simulink model "Aero_UltraStick25e"  (R2016b)
settings: Solver=VariableStepAuto  StartTime=0.0  StopTime=10.0  RelTol=1e-3
undefined symbols (not defined in the file or in its folder): AC
libraries: simulink x1
(part 2 of 2)

== system Aero_UltraStick25e/Yaw Moment Coefficient/Cnr*b//(2V) ==
  In : Inport
  2V : Gain  Gain=2  SaturateOnIntegerOverflow=on  OutDataTypeStr=Inherit: Same as input  ParamDataTypeStr=Inherit: Same as input
  Bus Selector4 : BusSelector  OutputSignals=AngVel.r_rps,WindAxesParams.alpha_rad,WindAxesParams.beta_rad,WindAxesParams.Vs_mps
  Cnr : Product
  Cnr Lookup : Interpolation_n-D  Table=AC.Aero.Cn.r_dat.data  InternalRulePriority=Speed
  Cnr*b/(2V) : Product  Inputs=**/  SaturateOnIntegerOverflow=on  RndMeth=Zero  InputSameDT=on  OutDataTypeStr=Inherit: Same as first input
  Prelookup Alpha : PreLookup  BreakpointsData=AC.Aero.CL.alpha_dat.alpha  ExtrapMethod=Linear
  Prelookup Beta : PreLookup  BreakpointsData=AC.Aero.CL.alpha_dat.beta  ExtrapMethod=Linear
  Wing span : Constant  Value=AC.Geometry.b
  Out : Outport
  wires:
  Bus Selector4/1 -> Cnr/1  "<r_rps>"
  In/1 -> Bus Selector4/1
  Prelookup Beta/1 -> Cnr Lookup/3
  Prelookup Beta/2 -> Cnr Lookup/4
  Prelookup Alpha/1 -> Cnr Lookup/1
  Bus Selector4/3 -> Prelookup Beta/1  "<beta_rad>"
  Bus Selector4/2 -> Prelookup Alpha/1  "<alpha_rad>"
  Prelookup Alpha/2 -> Cnr Lookup/2
  Cnr Lookup/1 -> Cnr/2
  2V/1 -> Cnr*b/(2V)/3
  Wing span/1 -> Cnr*b/(2V)/2
  Cnr/1 -> Cnr*b/(2V)/1
  Bus Selector4/4 -> 2V/1  "<Vs_mps>"
  Cnr*b/(2V)/1 -> Out/1

== system Aero_UltraStick25e/Lift Coefficient/CLq*c//(2V)/CLq ==
  In : Inport
  Bus Selector4 : BusSelector  OutputSignals=AngVel.q_rps,WindAxesParams.alpha_rad,WindAxesParams.beta_rad
  CLq : Product
  CLq Lookup : Interpolation_n-D  Table=AC.Aero.CL.q_dat.data  InternalRulePriority=Speed
  Prelookup Alpha : PreLookup  BreakpointsData=AC.Aero.CL.alpha_dat.alpha  ExtrapMethod=Linear
  Prelookup Beta : PreLookup  BreakpointsData=AC.Aero.CL.alpha_dat.beta  ExtrapMethod=Linear
  Out : Outport
  wires:
  CLq/1 -> Out/1
  CLq Lookup/1 -> CLq/2
  Prelookup Alpha/2 -> CLq Lookup/2
  Bus Selector4/2 -> Prelookup Alpha/1  "<alpha_rad>"
  Bus Selector4/3 -> Prelookup Beta/1  "<beta_rad>"
  Prelookup Alpha/1 -> CLq Lookup/1
  Prelookup Beta/2 -> CLq Lookup/4
  Prelookup Beta/1 -> CLq Lookup/3
  In/1 -> Bus Selector4/1
  Bus Selector4/1 -> CLq/1  "<q_rps>"
